simulink model "sf_spectrum_analyzer"  (Simulink 7.6)
settings: Solver=ode5  StartTime=0.0  StopTime=Inf  FixedStep=1e-4  MaxStep=1e-4  RelTol=1e-3
settings Model: Creator=The MathWorks Inc.
settings DataIOCC: LimitDataPoints=off
settings OptimizationCC: InitFltsAndDblsToZero=on  EfficientMapNaN2IntZero=off  OptimizeModelRefInitCode=on  LifeSpan=1
settings DebuggingCC: StrictBusMsg=Warning
settings SFSimCC: SimParseCustomCode=off
settings RTWCC: SystemTargetFile=ert.tlc  TemplateMakefile=ert_default_tmf  Description=Real-Time Workshop Embedded Coder (no auto configuration)  GenerateReport=on  ProcessScript=ert_make_rtw_hook  IncludeHyperlinkInReport=on  LaunchReport=on  GenerateTraceInfo=on  GenerateTraceReport=on  GenerateTraceReportSl=on  GenerateTraceReportSf=on  GenerateTraceReportEml=on
settings CodeAppCC: IgnoreCustomStorageClasses=off
settings ERTTargetCC: MultiwordLength=2048  GenerateSampleERTMain=on  SupportContinuousTime=on  InlinedParameterPlacement=NonHierarchical  ERTCustomFileTemplate=example_file_process.tlc  ConvertIfToSwitch=off

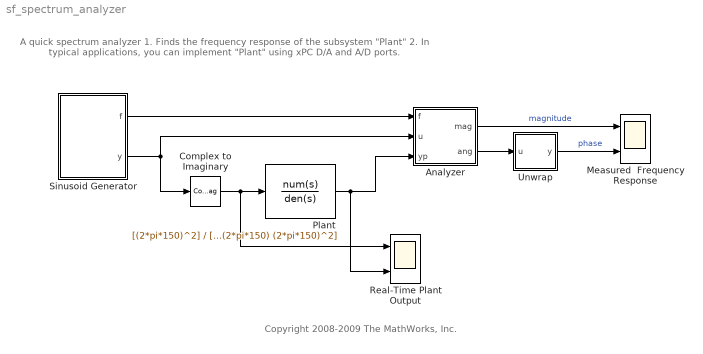
== system sf_spectrum_analyzer ==
  note: A quick spectrum analyzer
      | 1. Finds the frequency response of the subsystem "Plant"
      | 2. In typical applications, you can implement "Plant" using
      |     xPC D/A and A/D ports.
  note: Copyright 2008-2009 The MathWorks, Inc.
  Analyzer : Stateflow chart  TreatAsAtomicUnit=on
  Complex to Imaginary : ComplexToRealImag  Output=Imag
  Measured  Frequency Response : Scope  NumInputPorts=2
      settings: YMin=0~-4  YMax=1.8~0
  Plant : TransferFcn  Numerator=[(2*pi*150)^2]  Denominator=[1 2*0.3*(2*pi*150) (2*pi*150)^2]
  Real-Time Plant Output : Scope  NumInputPorts=2
      settings: YMin=0~-1.5  YMax=1.8~5
  Sinusoid Generator : Subsystem  TreatAsAtomicUnit=on  mask{fstart=10, fstop=1000, fstep=10, delay=0.2}
      mask prompts: fstart "Initial frequency"; fstop "Stop frequency"; fstep "Step frequency"; delay "Delay at each frequency"
      mask help: Outputs a signal with constantly increasing frequency
  Unwrap : Stateflow chart  TreatAsAtomicUnit=on
  wires:
  Complex to Imaginary/1 -> Plant/1, Real-Time Plant Output/1
  Plant/1 -> Analyzer/3(yp), Real-Time Plant Output/2
  Analyzer/1(mag) -> Measured  Frequency Response/1  "magnitude"
  Analyzer/2(ang) -> Unwrap/1(u)
  Sinusoid Generator/2(y) -> Complex to Imaginary/1, Analyzer/2(u)
  Sinusoid Generator/1(f) -> Analyzer/1(f)
  Unwrap/1(y) -> Measured  Frequency Response/2  "phase"

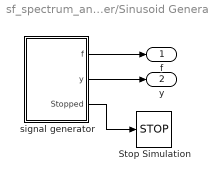
== system sf_spectrum_analyzer/Sinusoid Generator ==
  Stop Simulation : Stop
  signal generator : Stateflow chart  TreatAsAtomicUnit=on
  f : Outport
  y : Outport  Port=2
  wires:
  signal generator/2(y) -> y/1
  signal generator/1(f) -> f/1
  signal generator/3(Stopped) -> Stop Simulation/1

== stateflow chart Sinusoid Generator/signal generator ==
  state A
    du:
    computey(temporalCount(sec));
  state Stopped
    y = 0;
  A -> (junction 6) : [after(delay,sec) && imag(yprev)*imag(y) <= 0 && imag(y) > 0]
      | {
      | f += fstep;
      | }
  (default) -> A : {f = fstart;}
  (junction 6) -> Stopped [order 1] : [f > fstop]
  (junction 6) -> A [order 2]
  data: t function_input double; delay parameter double; f output double; y output double; yprev local double; fstep parameter double; fstart parameter double; fstop parameter double; Stopped output boolean
  function computey(t):
    | function computey(t)
    | yprev = y;
    | y = exp(2*pi*f*t*1j);

== stateflow chart Analyzer ==
  state A
    en:
    y = 0; yn = 0;
    du:
    y += u*yp;
    yn += u*imag(u);
  A -> A : [hasChanged(f)]
      | {
      | computeOutputs();
      | }
  data: f input double; mag output double; ang output double; u input double; y local double; yn local double; yp input double
  function computeOutputs:
    | function computeOutputs
    | 
    | mag = abs(y)/abs(yn);
    | ang = -angle(y) + pi/2;

== stateflow chart Unwrap ==
  state A
    (default) -> (junction 36)
    A -> (junction 36) [order 1]
    (junction 36) -> (junction 37) : {
        | y = u + offset;
        | yprev = y;
        | }
  (junction 35) -> A [order 2] : [u+offset-yprev > PI]
      | { offset -= 2*PI; }
  A -> (junction 35) [order 1]
  (junction 35) -> A [order 1] : [u+offset-yprev < -PI]
      | { offset += 2*PI;}
  data: PI constant double =pi; offset local double; u input double; y output double; yprev local double
